simulink model "PID"  (R2018b)
settings: Solver=VariableStepAuto  StartTime=0.0  StopTime=10.0  RelTol=1e-3
values from neighbouring files (symbols this model uses):
  c = eRange/2-m*maxLight    (= -143.181818182)    [lightVsError.m]
  m = eRange/(maxLight-minLight)    (= 0.272727272727)    [lightVsError.m]
undefined symbols (not defined in the file or in its folder): KD, KI, KP
settings Model: Creator=Brus  LastModifiedBy=Brus

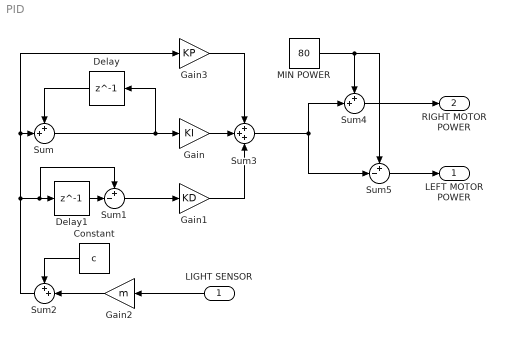
== system PID ==
  LIGHT SENSOR : Inport
  Constant : Constant  Value=c
  Delay : Delay  DelayLength=1
  Delay1 : Delay  DelayLength=1
  Gain : Gain  Gain=KI
  Gain1 : Gain  Gain=KD
  Gain2 : Gain  Gain=m
  Gain3 : Gain  Gain=KP
  MIN POWER : Constant  Value=80
  Sum : Sum  Inputs=++|
  Sum1 : Sum  Inputs=+-|
  Sum2 : Sum  Inputs=++|
  Sum3 : Sum  Inputs=+++
  Sum4 : Sum  Inputs=++|
  Sum5 : Sum  Inputs=+-|
  LEFT MOTOR POWER : Outport
  RIGHT MOTOR POWER : Outport  Port=2
  wires:
  Delay/1 -> Sum/1
  Delay1/1 -> Sum1/2
  Sum2/1 -> Sum1/1, Delay1/1, Sum/2, Gain3/1
  Sum1/1 -> Gain1/1
  Gain2/1 -> Sum2/2
  Constant/1 -> Sum2/1
  LIGHT SENSOR/1 -> Gain2/1
  Gain/1 -> Sum3/2
  Gain3/1 -> Sum3/1
  Gain1/1 -> Sum3/3
  Sum3/1 -> Sum5/2, Sum4/2
  MIN POWER/1 -> Sum4/1, Sum5/1
  Sum4/1 -> RIGHT MOTOR POWER/1
  Sum5/1 -> LEFT MOTOR POWER/1
  Sum/1 -> Delay/1, Gain/1
